simulink model "Ports_Subsystems_Lib"  (R2020b)
settings: Solver=FixedStepDiscrete  StartTime=0.0  StopTime=10.0  FixedStep=0.01  RelTol=1e-3
libraries: simulink x5
settings Model: Creator=Emiliano  LastModifiedBy=Emiliano
settings OptimizationCC: DefaultParameterBehavior=Inlined  UseDivisionForNetSlopeComputation=on  GainParamInheritBuiltInType=on  UseFloatMulNetSlope=on  InlineInvariantSignals=on  PassReuseOutputArgsAs=Individual arguments  ZeroExternalMemoryAtStartup=off  ZeroInternalMemoryAtStartup=off  NoFixptDivByZeroProtection=on  EfficientFloat2IntCast=on  LifeSpan=1  OptimizeBlockOrder=speed  DifferentSizesBufferReuse=on  EfficientTunableParamExpr=on
settings DebuggingCC: ParameterTunabilityLossMsg=error
settings HardwareCC: ProdLongLongMode=on
settings SFSimCC: MATLABDynamicMemAlloc=off
settings RTWCC: Description=Embedded Coder  SystemTargetFile=ert.tlc  TemplateMakefile=ert_default_tmf
settings CodeAppCC: ForceParamTrailComments=on  IgnoreCustomStorageClasses=off  OperatorAnnotations=on  SimulinkDataObjDesc=on  SFDataObjDesc=on  CustomSymbolStrGlobalVar=rt$N$M  CustomSymbolStrType=$N$M  CustomSymbolStrFcn=$N$M$F  CustomSymbolStrMacro=$N$M  InsertBlockDesc=on
settings ERTTargetCC: TargetLangStandard=C99 (ISO)  GenerateSampleERTMain=on  IncludeMdlTerminateFcn=off  CombineSignalStateStructs=on  SupportComplex=off  SupportNonInlinedSFcns=on  InlinedParameterPlacement=NonHierarchical  ERTCustomFileTemplate=example_file_process.tlc  ERTFilePackagingFormat=CompactWithDataFile

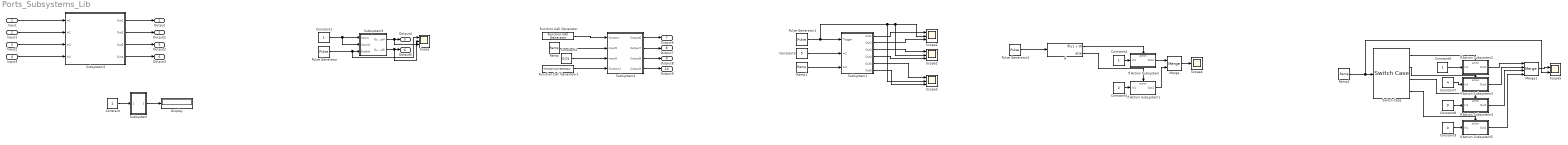
== system Ports_Subsystems_Lib ==
  Input : Inport
  Input1 : Inport  Port=2
  Input2 : Inport  Port=3
  Input3 : Inport  Port=4
  Constant{,1,4,6} (4 alike) : Constant
  Constant2 : Constant  Value=0.01
  Constant3 : Constant  Value=5
  Constant5 : Constant  Value=2
  Constant7 : Constant  Value=4
  Constant8 : Constant  Value=9
  Constant9 : Constant  Value=0
  Display : Display
  Function-Call Generator : simulink/Ports & Subsystems/Function-Call Generator  sample_time=1  numberOfIterations=5  DisallowWideOutput=off
  Function-Call Generator1 : simulink/Ports & Subsystems/Function-Call Generator  sample_time=1  numberOfIterations=10  DisallowWideOutput=off
  If : If
  If Action Subsystem : Subsystem  TreatAsAtomicUnit=on
  If Action Subsystem1 : Subsystem  TreatAsAtomicUnit=on
  If Action Subsystem2 : Subsystem  TreatAsAtomicUnit=on
  If Action Subsystem3 : Subsystem  TreatAsAtomicUnit=on
  If Action Subsystem4 : Subsystem  TreatAsAtomicUnit=on
  If Action Subsystem5 : Subsystem  TreatAsAtomicUnit=on
  Merge : Merge
  Merge1 : Merge  Inputs=4
  Pulse Generator : DiscretePulseGenerator  PulseType=Time based  Period=1  PulseWidth=50
  Pulse Generator1 : DiscretePulseGenerator  PulseType=Time based  Period=1  PulseWidth=50
  Pulse Generator2 : DiscretePulseGenerator  PulseType=Time based  Amplitude=2  Period=1  PulseWidth=50
  Ramp : simulink/Sources/Ramp  slope=1  start=0  InitialOutput=0
  Ramp1 : simulink/Sources/Ramp  slope=1  start=0  InitialOutput=0
  Ramp2 : simulink/Sources/Ramp  slope=1  start=0  InitialOutput=0
  Scope{,1..3} (4 alike) : Scope  NumInputPorts=3
  Scope4 : Scope
  Scope5 : Scope  NumInputPorts=2
  Subsystem : Subsystem  mask{Shifting_Value=5, Scaling_Value=0, Min_Value=[], Max_Value=[], Parameter5=1}
      mask prompts: Shifting_Value "Shifting Value"; Scaling_Value "Scaling Value"; Min_Value "Min"; Max_Value "Max"; Parameter5 "Combo options"
      mask TypeOptions Parameter5: 1 | 2 | 3 | 4 | 5
      mask DialogControl DescTextVar Prompt: This mask shifts and scales an input
      mask DialogControl Container4 Prompt: Main
      mask DialogControl Container7 Prompt: Signal
  Subsystem1 : Subsystem
  Subsystem2 : Subsystem
  Subsystem3 : Subsystem
  Subsystem4 : Subsystem
  Switch Case : SwitchCase  CaseConditions={1,2,3}
  Output : Outport
  Output1 : Outport  Port=2
  Output2 : Outport  Port=3
  Output3 : Outport  Port=4
  Output4 : Outport  Port=5
  Output5 : Outport  Port=6
  Output6 : Outport  Port=7
  Output7 : Outport  Port=8
  Output8 : Outport  Port=9
  Output9 : Outport  Port=10
  wires:
  Input/1 -> Subsystem2/1(In1)
  Input1/1 -> Subsystem2/2(In2)
  Input2/1 -> Subsystem2/3(In3)
  Input3/1 -> Subsystem2/4(In4)
  Subsystem2/1(Out1) -> Output/1
  Subsystem2/2(Out2) -> Output1/1
  Subsystem2/3(Out3) -> Output2/1
  Subsystem2/4(Out4) -> Output3/1
  Constant/1 -> Subsystem/1(In1)
  Subsystem/1(Out1) -> Display/1
  Constant1/1 -> Subsystem3/2(Inport1), Subsystem3/1(Inport)
  Subsystem3/1(Output4) -> Scope/1, Output4/1
  Subsystem3/2(Output5) -> Scope/2, Output5/1
  Pulse Generator/1 -> Scope/3, Subsystem3/3(Enable)
  Subsystem4/1(Output6) -> Output6/1
  Subsystem4/4(Output9) -> Output9/1
  Subsystem4/3(Output8) -> Output8/1
  Subsystem4/2(Output7) -> Output7/1
  Constant2/1 -> Subsystem4/3(Input6)
  Ramp/1 -> Subsystem4/2(Input5)
  Function-Call Generator/1 -> Subsystem4/1(function)
  Function-Call Generator1/1 -> Subsystem4/4(function1)
  Pulse Generator1/1 -> Scope3/2, Scope2/2, Scope1/2, Subsystem1/1(Trigger)
  Constant3/1 -> Subsystem1/2(In2)
  Ramp1/1 -> Subsystem1/3(In3)
  Subsystem1/1(Out1) -> Scope1/1
  Subsystem1/2(Out2) -> Scope1/3
  Subsystem1/3(Out3) -> Scope2/1
  Subsystem1/4(Out4) -> Scope2/3
  Subsystem1/5(Out5) -> Scope3/1
  Subsystem1/6(Out6) -> Scope3/3
  Constant4/1 -> If Action Subsystem/1(In1)
  If Action Subsystem/1(Out1) -> Merge/1
  If/1 -> If Action Subsystem/Action
  If/2 -> If Action Subsystem1/Action
  Constant5/1 -> If Action Subsystem1/1(In1)
  If Action Subsystem1/1(Out1) -> Merge/2
  Merge/1 -> Scope4/1
  Pulse Generator2/1 -> If/1
  Ramp2/1 -> Scope5/2, Switch Case/1
  Switch Case/1 -> If Action Subsystem2/Action
  Switch Case/2 -> If Action Subsystem3/Action
  Switch Case/3 -> If Action Subsystem4/Action
  Switch Case/4 -> If Action Subsystem5/Action
  Constant6/1 -> If Action Subsystem2/1(In1)
  Constant9/1 -> If Action Subsystem5/1(In1)
  Constant8/1 -> If Action Subsystem4/1(In1)
  Constant7/1 -> If Action Subsystem3/1(In1)
  If Action Subsystem2/1(Out1) -> Merge1/1
  If Action Subsystem3/1(Out1) -> Merge1/2
  If Action Subsystem4/1(Out1) -> Merge1/3
  If Action Subsystem5/1(Out1) -> Merge1/4
  Merge1/1 -> Scope5/1

== system Ports_Subsystems_Lib/If Action Subsystem ==
  In1 : Inport
  Action Port : ActionPort  ActionPortLabel=if(u1 > 0)
  Out1 : Outport
  wires:
  In1/1 -> Out1/1

== system Ports_Subsystems_Lib/If Action Subsystem1 ==
  In1 : Inport
  Action Port : ActionPort  ActionPortLabel=else
  Out1 : Outport
  wires:
  In1/1 -> Out1/1

== system Ports_Subsystems_Lib/If Action Subsystem2 ==
  In1 : Inport
  Action Port : ActionPort  ActionPortLabel=case [ 1 ]:
  Out1 : Outport
  wires:
  In1/1 -> Out1/1

== system Ports_Subsystems_Lib/If Action Subsystem3 ==
  In1 : Inport
  Action Port : ActionPort  ActionPortLabel=case [ 2 ]:
  Out1 : Outport
  wires:
  In1/1 -> Out1/1

== system Ports_Subsystems_Lib/If Action Subsystem4 ==
  In1 : Inport
  Action Port : ActionPort  ActionPortLabel=case [ 3 ]:
  Out1 : Outport
  wires:
  In1/1 -> Out1/1

== system Ports_Subsystems_Lib/If Action Subsystem5 ==
  In1 : Inport
  Action Port : ActionPort  ActionPortLabel=default:
  Out1 : Outport
  wires:
  In1/1 -> Out1/1

== system Ports_Subsystems_Lib/Subsystem ==
  In1 : Inport
  Add : Sum
  Constant : Constant  Value=Shifting_Value
  Multiply : Gain  Gain=Scaling_Value
  Out1 : Outport
  wires:
  Constant/1 -> Add/2
  Multiply/1 -> Out1/1
  Add/1 -> Multiply/1
  In1/1 -> Add/1

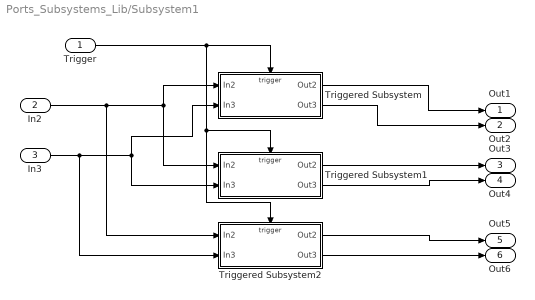
== system Ports_Subsystems_Lib/Subsystem1 ==
  Trigger : Inport
  In2 : Inport  Port=2
  In3 : Inport  Port=3
  Triggered Subsystem : Subsystem  TreatAsAtomicUnit=on
  Triggered Subsystem1 : Subsystem  TreatAsAtomicUnit=on
  Triggered Subsystem2 : Subsystem  TreatAsAtomicUnit=on
  Out1 : Outport
  Out2 : Outport  Port=2
  Out3 : Outport  Port=3
  Out4 : Outport  Port=4
  Out5 : Outport  Port=5
  Out6 : Outport  Port=6
  wires:
  In3/1 -> Triggered Subsystem2/2(In3), Triggered Subsystem1/2(In3), Triggered Subsystem/2(In3)
  Trigger/1 -> Triggered Subsystem2/Trigger, Triggered Subsystem1/Trigger, Triggered Subsystem/Trigger
  Triggered Subsystem1/2(Out3) -> Out4/1
  In2/1 -> Triggered Subsystem2/1(In2), Triggered Subsystem1/1(In2), Triggered Subsystem/1(In2)
  Triggered Subsystem1/1(Out2) -> Out3/1
  Triggered Subsystem2/2(Out3) -> Out6/1
  Triggered Subsystem/1(Out2) -> Out1/1
  Triggered Subsystem2/1(Out2) -> Out5/1
  Triggered Subsystem/2(Out3) -> Out2/1

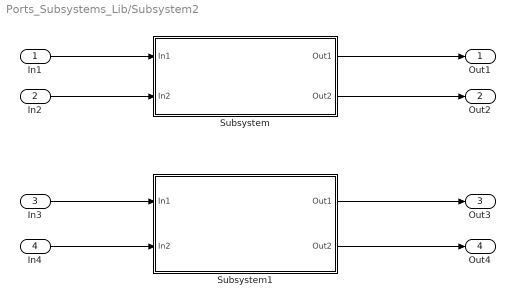
== system Ports_Subsystems_Lib/Subsystem2 ==
  In1 : Inport
  In2 : Inport  Port=2
  In3 : Inport  Port=3
  In4 : Inport  Port=4
  Subsystem : Subsystem  TreatAsAtomicUnit=on
  Subsystem1 : Subsystem
  Out1 : Outport
  Out2 : Outport  Port=2
  Out3 : Outport  Port=3
  Out4 : Outport  Port=4
  wires:
  In1/1 -> Subsystem/1(In1)
  In2/1 -> Subsystem/2(In2)
  Subsystem1/2(Out2) -> Out4/1
  Subsystem/1(Out1) -> Out1/1
  Subsystem/2(Out2) -> Out2/1
  In3/1 -> Subsystem1/1(In1)
  In4/1 -> Subsystem1/2(In2)
  Subsystem1/1(Out1) -> Out3/1

== system Ports_Subsystems_Lib/Subsystem3 ==
  Inport : Inport
  Inport1 : Inport  Port=2
  Enable : Inport  Port=3
  Subsystem1 : Subsystem
  Output4 : Outport
  Output5 : Outport  Port=2
  wires:
  Enable/1 -> Subsystem1/Enable
  Subsystem1/1(Out1) -> Output4/1
  Inport/1 -> Subsystem1/1(In1)
  Inport1/1 -> Subsystem1/2(In2)
  Subsystem1/2(Out2) -> Output5/1

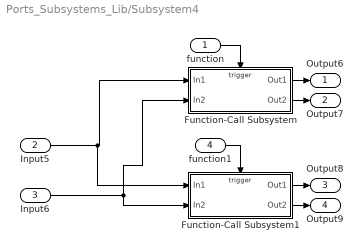
== system Ports_Subsystems_Lib/Subsystem4 ==
  function : Inport
  Input5 : Inport  Port=2
  Input6 : Inport  Port=3
  function1 : Inport  Port=4
  Function-Call Subsystem : Subsystem  TreatAsAtomicUnit=on
  Function-Call Subsystem1 : Subsystem  TreatAsAtomicUnit=on
  Output6 : Outport
  Output7 : Outport  Port=2
  Output8 : Outport  Port=3
  Output9 : Outport  Port=4
  wires:
  Function-Call Subsystem1/2(Out2) -> Output9/1
  Function-Call Subsystem1/1(Out1) -> Output8/1
  Input6/1 -> Function-Call Subsystem/2(In2), Function-Call Subsystem1/2(In2)
  Input5/1 -> Function-Call Subsystem1/1(In1), Function-Call Subsystem/1(In1)
  function1/1 -> Function-Call Subsystem1/Trigger
  function/1 -> Function-Call Subsystem/Trigger
  Function-Call Subsystem/1(Out1) -> Output6/1
  Function-Call Subsystem/2(Out2) -> Output7/1

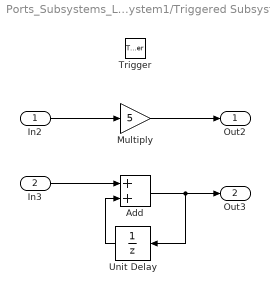
== system Ports_Subsystems_Lib/Subsystem1/Triggered Subsystem ==
  In2 : Inport
  In3 : Inport  Port=2
  Trigger : TriggerPort  VariantControl=Variant
  Add : Sum
  Multiply : Gain  Gain=5
  Unit Delay : UnitDelay  SampleTime=-1  HasFrameUpgradeWarning=on
  Out2 : Outport
  Out3 : Outport  Port=2
  wires:
  Multiply/1 -> Out2/1
  Add/1 -> Out3/1, Unit Delay/1
  Unit Delay/1 -> Add/2
  In3/1 -> Add/1
  In2/1 -> Multiply/1

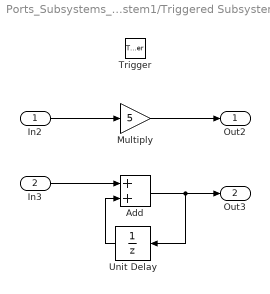
== system Ports_Subsystems_Lib/Subsystem1/Triggered Subsystem1 ==
  In2 : Inport
  In3 : Inport  Port=2
  Trigger : TriggerPort  TriggerType=falling  VariantControl=Variant
  Add : Sum
  Multiply : Gain  Gain=5
  Unit Delay : UnitDelay  SampleTime=-1  HasFrameUpgradeWarning=on
  Out2 : Outport
  Out3 : Outport  Port=2
  wires:
  Multiply/1 -> Out2/1
  Add/1 -> Out3/1, Unit Delay/1
  Unit Delay/1 -> Add/2
  In3/1 -> Add/1
  In2/1 -> Multiply/1

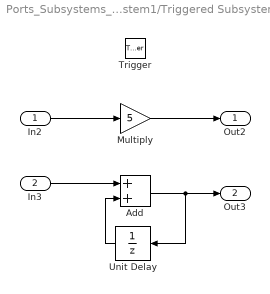
== system Ports_Subsystems_Lib/Subsystem1/Triggered Subsystem2 ==
  In2 : Inport
  In3 : Inport  Port=2
  Trigger : TriggerPort  TriggerType=either  VariantControl=Variant
  Add : Sum
  Multiply : Gain  Gain=5
  Unit Delay : UnitDelay  SampleTime=-1  HasFrameUpgradeWarning=on
  Out2 : Outport
  Out3 : Outport  Port=2
  wires:
  Multiply/1 -> Out2/1
  Add/1 -> Out3/1, Unit Delay/1
  Unit Delay/1 -> Add/2
  In3/1 -> Add/1
  In2/1 -> Multiply/1

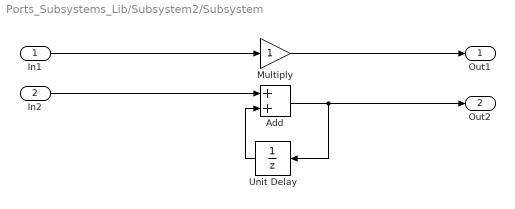
== system Ports_Subsystems_Lib/Subsystem2/Subsystem ==
  In1 : Inport
  In2 : Inport  Port=2
  Add : Sum
  Multiply : Gain
  Unit Delay : UnitDelay  SampleTime=-1  HasFrameUpgradeWarning=on
  Out1 : Outport
  Out2 : Outport  Port=2
  wires:
  Unit Delay/1 -> Add/2
  Add/1 -> Out2/1, Unit Delay/1
  In1/1 -> Multiply/1
  In2/1 -> Add/1
  Multiply/1 -> Out1/1

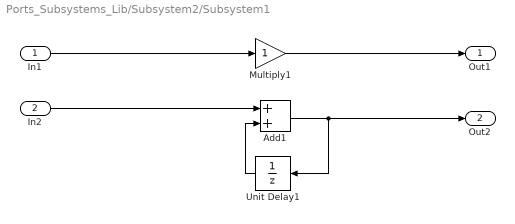
== system Ports_Subsystems_Lib/Subsystem2/Subsystem1 ==
  In1 : Inport
  In2 : Inport  Port=2
  Add1 : Sum
  Multiply1 : Gain
  Unit Delay1 : UnitDelay  SampleTime=-1  HasFrameUpgradeWarning=on
  Out1 : Outport
  Out2 : Outport  Port=2
  wires:
  In2/1 -> Add1/1
  Unit Delay1/1 -> Add1/2
  Add1/1 -> Out2/1, Unit Delay1/1
  In1/1 -> Multiply1/1
  Multiply1/1 -> Out1/1

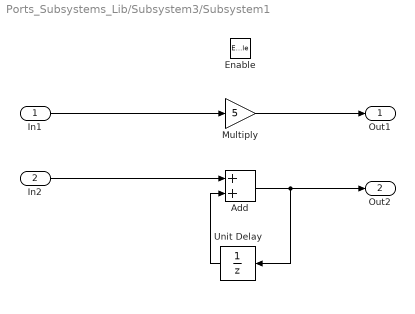
== system Ports_Subsystems_Lib/Subsystem3/Subsystem1 ==
  In1 : Inport
  In2 : Inport  Port=2
  Enable : EnablePort  StatesWhenEnabling=reset
  Add : Sum
  Multiply : Gain  Gain=5
  Unit Delay : UnitDelay  SampleTime=-1  HasFrameUpgradeWarning=on
  Out1 : Outport
  Out2 : Outport  Port=2
  wires:
  Add/1 -> Out2/1, Unit Delay/1
  In2/1 -> Add/1
  Unit Delay/1 -> Add/2
  Multiply/1 -> Out1/1
  In1/1 -> Multiply/1

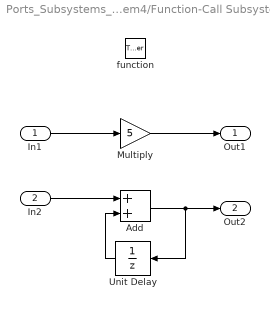
== system Ports_Subsystems_Lib/Subsystem4/Function-Call Subsystem ==
  In1 : Inport
  In2 : Inport  Port=2
  function : TriggerPort  TriggerType=function-call  VariantControl=Variant
  Add : Sum
  Multiply : Gain  Gain=5
  Unit Delay : UnitDelay  SampleTime=-1  HasFrameUpgradeWarning=on
  Out1 : Outport
  Out2 : Outport  Port=2
  wires:
  In1/1 -> Multiply/1
  Add/1 -> Out2/1, Unit Delay/1
  In2/1 -> Add/1
  Unit Delay/1 -> Add/2
  Multiply/1 -> Out1/1

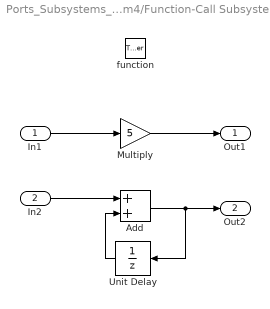
== system Ports_Subsystems_Lib/Subsystem4/Function-Call Subsystem1 ==
  In1 : Inport
  In2 : Inport  Port=2
  function : TriggerPort  TriggerType=function-call  VariantControl=Variant  StatesWhenEnabling=reset
  Add : Sum
  Multiply : Gain  Gain=5
  Unit Delay : UnitDelay  SampleTime=-1  HasFrameUpgradeWarning=on
  Out1 : Outport
  Out2 : Outport  Port=2
  wires:
  In1/1 -> Multiply/1
  Add/1 -> Out2/1, Unit Delay/1
  In2/1 -> Add/1
  Unit Delay/1 -> Add/2
  Multiply/1 -> Out1/1
